simulink model "Asw_PMSMCtrl"  (R2023a)
settings: Solver=FixedStepDiscrete  StartTime=0.0  StopTime=10.0  RelTol=1e-3  EnableMultiTasking=on
values from neighbouring files (symbols this model uses):
  Hw_Par_fVdc = Simulink.Parameter    [Asw_PMSMCtrl_Parameters.m]
  Mt_Par_fNp = Simulink.Parameter    [Asw_PMSMCtrl_Parameters.m]
undefined symbols (not defined in the file or in its folder): Sw_Par_fTs
libraries: mcbcontrolslib x5
settings Model: Creator=62555  LastModifiedBy=62555
settings OptimizationCC: DefaultUnderspecifiedDataType=single  EnhancedBackFolding=on  PassReuseOutputArgsAs=Individual arguments  ZeroExternalMemoryAtStartup=off  ZeroInternalMemoryAtStartup=off  MaxStackSize=64  OptimizeBlockOrder=speed  DifferentSizesBufferReuse=on  OptimizationCustomize=off  EfficientTunableParamExpr=on
settings DebuggingCC: ParameterOverflowMsg=none  ParameterUnderflowMsg=error  ParameterTunabilityLossMsg=error
settings HardwareCC: ProdBitPerPointer=32  ProdBitPerSizeT=32  ProdBitPerPtrDiffT=32  ProdLargestAtomicInteger=Long  ProdLargestAtomicFloat=Double  ProdWordSize=32  ProdLongLongMode=on  ProdHWDeviceType=ARM Compatible->ARM Cortex
settings SFSimCC: MATLABDynamicMemAlloc=off
settings RTWCC: Description=Embedded Coder  SystemTargetFile=ert.tlc  HardwareBoard=STM32G4xx Based  TemplateMakefile=ert_default_tmf  GenerateReport=on  Toolchain=GNU Tools for ARM Embedded Processors  LaunchReport=on
settings CodeAppCC: ForceParamTrailComments=on  IgnoreCustomStorageClasses=off  OperatorAnnotations=on  SimulinkDataObjDesc=on  SFDataObjDesc=on  InsertBlockDesc=on
settings ERTTargetCC: TargetLangStandard=C99 (ISO)  CodeReplacementLibrary=ARM Cortex-M  ExtModeTransport=3  ExtModeStaticAlloc=on  ExtModeStaticAllocSize=2048  ExtModeMexFile=ext_xcp  ExtModeIntrfLevel=Level2 - Open

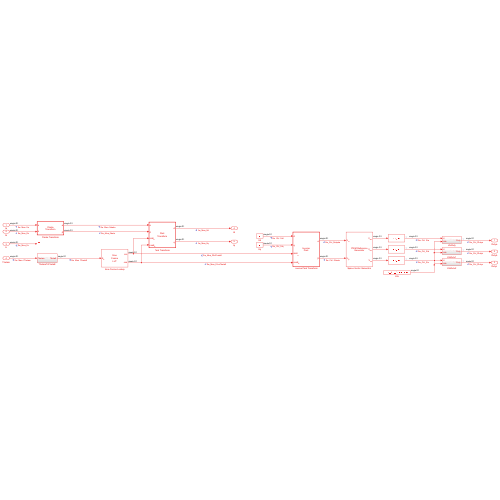
[thumbnail: Simulink's stored preview of the top-level diagram]
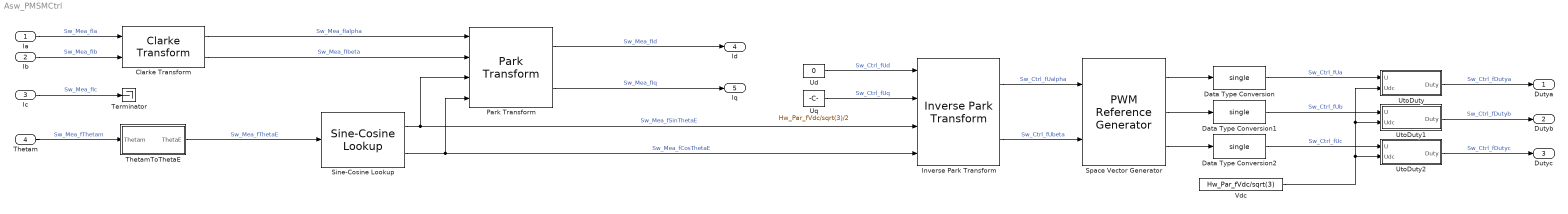
== system Asw_PMSMCtrl ==
  Ia : Inport
  Ib : Inport  Port=2
  Ic : Inport  Port=3
  Thetam : Inport  Port=4
  Clarke Transform : mcbcontrolslib/Clarke Transform  VariantControl=Variant2
  Data Type Conversion : DataTypeConversion  OutDataTypeStr=single  SaturateOnIntegerOverflow=off  RndMeth=Floor
  Data Type Conversion1 : DataTypeConversion  OutDataTypeStr=single  SaturateOnIntegerOverflow=off  RndMeth=Floor
  Data Type Conversion2 : DataTypeConversion  OutDataTypeStr=single  SaturateOnIntegerOverflow=off  RndMeth=Floor
  Inverse Park Transform : mcbcontrolslib/Inverse Park Transform  AxisAlignment=D-axis
  Park Transform : mcbcontrolslib/Park Transform  AxisAlignment=D-axis
  Sine-Cosine Lookup : mcbcontrolslib/Sine-Cosine Lookup  AngleInput=Radians  N_points=4095
  Space Vector Generator : mcbcontrolslib/PWM Reference Generator  inSignal=Valphabeta  modType=SVM: space vector modulation
  Terminator : Terminator
  ThetamToThetaE : Subsystem
  Ud : Constant  Value=0  OutDataTypeStr=single  SampleTime=Sw_Par_fTs
  Uq : Constant  Value=Hw_Par_fVdc/sqrt(3)/2  OutDataTypeStr=single  SampleTime=Sw_Par_fTs
  UtoDuty : Subsystem
  UtoDuty1 : Subsystem
  UtoDuty2 : Subsystem
  Vdc : Constant  Value=Hw_Par_fVdc/sqrt(3)  OutDataTypeStr=single  SampleTime=Sw_Par_fTs
  Dutya : Outport
  Dutyb : Outport  Port=2
  Dutyc : Outport  Port=3
  Id : Outport  Port=4
  Iq : Outport  Port=5
  wires:
  Clarke Transform/2 -> Park Transform/2  "Sw_Mea_fIbeta"
  Inverse Park Transform/1 -> Space Vector Generator/1  "Sw_Ctrl_fUalpha"
  Ud/1 -> Inverse Park Transform/1  "Sw_Ctrl_fUd"
  Uq/1 -> Inverse Park Transform/2  "Sw_Ctrl_fUq"
  Clarke Transform/1 -> Park Transform/1  "Sw_Mea_fIalpha"
  Ia/1 -> Clarke Transform/1  "Sw_Mea_fIa"
  Ib/1 -> Clarke Transform/2  "Sw_Mea_fIb"
  Sine-Cosine Lookup/1 -> Inverse Park Transform/3, Park Transform/3  "Sw_Mea_fSinThetaE"
  Inverse Park Transform/2 -> Space Vector Generator/2  "Sw_Ctrl_fUbeta"
  Ic/1 -> Terminator/1  "Sw_Mea_fIc"
  Park Transform/2 -> Iq/1  "Sw_Mea_fIq"
  Park Transform/1 -> Id/1  "Sw_Mea_fId"
  Thetam/1 -> ThetamToThetaE/1(Thetam)  "Sw_Mea_fThetam"
  Sine-Cosine Lookup/2 -> Park Transform/4, Inverse Park Transform/4  "Sw_Mea_fCosThetaE"
  ThetamToThetaE/1(ThetaE) -> Sine-Cosine Lookup/1  "Sw_Mea_fThetaE"
  Space Vector Generator/1 -> Data Type Conversion/1
  Space Vector Generator/2 -> Data Type Conversion1/1
  Space Vector Generator/3 -> Data Type Conversion2/1
  Data Type Conversion/1 -> UtoDuty/1(U)  "Sw_Ctrl_fUa"
  Data Type Conversion1/1 -> UtoDuty1/1(U)  "Sw_Ctrl_fUb"
  Data Type Conversion2/1 -> UtoDuty2/1(U)  "Sw_Ctrl_fUc"
  UtoDuty/1(Duty) -> Dutya/1  "Sw_Ctrl_fDutya"
  UtoDuty1/1(Duty) -> Dutyb/1  "Sw_Ctrl_fDutyb"
  UtoDuty2/1(Duty) -> Dutyc/1  "Sw_Ctrl_fDutyc"
  Vdc/1 -> UtoDuty2/2(Udc), UtoDuty1/2(Udc), UtoDuty/2(Udc)

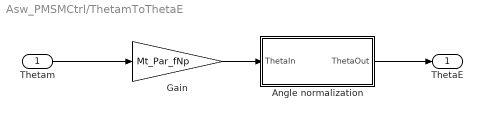
== system Asw_PMSMCtrl/ThetamToThetaE ==
  Thetam : Inport
  Angle normalization : MATLAB Function  TreatAsAtomicUnit=on
  Gain : Gain  Gain=Mt_Par_fNp
  ThetaE : Outport
  wires:
  Gain/1 -> Angle normalization/1(ThetaIn)
  Thetam/1 -> Gain/1
  Angle normalization/1(ThetaOut) -> ThetaE/1

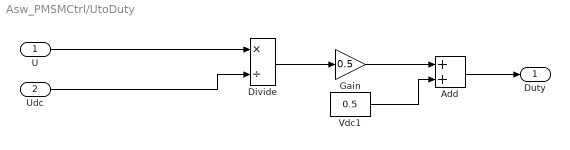
== system Asw_PMSMCtrl/UtoDuty ==
  U : Inport
  Udc : Inport  Port=2
  Add : Sum
  Divide : Product  Inputs=*/
  Gain : Gain  Gain=0.5
  Vdc1 : Constant  Value=0.5  OutDataTypeStr=single  SampleTime=Sw_Par_fTs
  Duty : Outport
  wires:
  Divide/1 -> Gain/1
  Gain/1 -> Add/1
  Vdc1/1 -> Add/2
  U/1 -> Divide/1
  Add/1 -> Duty/1
  Udc/1 -> Divide/2

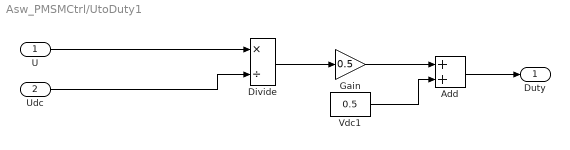
== system Asw_PMSMCtrl/UtoDuty1 ==
  U : Inport
  Udc : Inport  Port=2
  Add : Sum
  Divide : Product  Inputs=*/
  Gain : Gain  Gain=0.5
  Vdc1 : Constant  Value=0.5  OutDataTypeStr=single  SampleTime=Sw_Par_fTs
  Duty : Outport
  wires:
  Divide/1 -> Gain/1
  Gain/1 -> Add/1
  Vdc1/1 -> Add/2
  U/1 -> Divide/1
  Add/1 -> Duty/1
  Udc/1 -> Divide/2

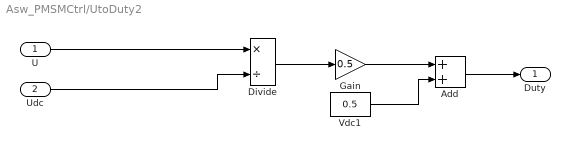
== system Asw_PMSMCtrl/UtoDuty2 ==
  U : Inport
  Udc : Inport  Port=2
  Add : Sum
  Divide : Product  Inputs=*/
  Gain : Gain  Gain=0.5
  Vdc1 : Constant  Value=0.5  OutDataTypeStr=single  SampleTime=Sw_Par_fTs
  Duty : Outport
  wires:
  Divide/1 -> Gain/1
  Gain/1 -> Add/1
  Vdc1/1 -> Add/2
  U/1 -> Divide/1
  Add/1 -> Duty/1
  Udc/1 -> Divide/2

== matlab function Asw_PMSMCtrl/ThetamToThetaE/Angle normalization ==
  data: ThetaIn input; ThetaOut output
function ThetaOut = fcn(ThetaIn)

Theta = ThetaIn;

while(Theta > single(2*pi))
    Theta = Theta - single(2*pi);
end

while(Theta < single(0))
    Theta = Theta + single(2*pi);
end

ThetaOut = Theta;
